simulink library "Pipe_BiFlow"  (R2018b)
settings: Solver=ode45  StartTime=0.0  StopTime=10.0  RelTol=1e-3  EnableMultiTasking=on
undefined symbols (not defined in the file): path_carnot
libraries: carnot x5
settings Model: Creator=drhf  LastModifiedBy=P41573
settings DataIOCC: LimitDataPoints=on  SaveFormat=Array  SignalLoggingSaveFormat=ModelDataLogs
settings OptimizationCC: ExpressionDepthLimit=2147483647  LifeSpan=inf
settings DebuggingCC: UnderspecifiedInitializationDetection=Classic  MergeDetectMultiDrivingBlocksExec=none  SolverPrmCheckMsg=warning  FcnCallInpInsideContextMsg=warning  StateNameClashWarn=warning  SFUnexpectedBacktrackingDiag=warning  SFNoUnconditionalDefaultTransitionDiag=warning  SFExecutionAtInitializationDiag=none
settings HardwareCC: ProdBitPerPointer=32  ProdBitPerSizeT=32  ProdBitPerPtrDiffT=32  ProdLargestAtomicFloat=None  ProdIntDivRoundTo=Undefined  ProdEndianess=Unspecified  ProdWordSize=32  ProdHWDeviceType=32-bit Generic
settings ModelReferenceCC: PropagateSignalLabelsOutOfModel=off
settings SFSimCC: SimUseLocalCustomCode=off
settings RTWCC: RTWUseLocalCustomCode=off
settings CodeAppCC: StateflowObjectComments=on
settings GRTTargetCC: TargetLangStandard=C89/C90 (ANSI)  GeneratePreprocessorConditionals=Disable all  CombineOutputUpdateFcns=off  GRTInterface=on
settings ConfigComp: CovMetricSettings=dw  CovHtmlReporting=on  CovSaveCumulativeToWorkspaceVar=on  CovSaveSingleToWorkspaceVar=on  CovExternalEMLEnable=off

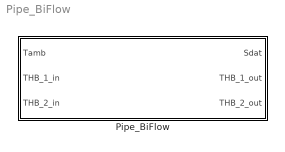
== system Pipe_BiFlow ==
  Pipe_BiFlow : Subsystem  mask(Pipe Biflow){t0=20, hgt=1273.2395, stgtype=1, tini=[20 20 20 20 20 20 20 20 20 20], mpts=[1 2 3 4 5 6 7 8 9 10], PathName=fullfile(path_carnot('libsl'),'Hydraulics','Pipe_BiFlow','parameter_set'), FileName='PipeBF_set1.mat', userPath=off, userParam=off, uwall=1, ubot=0, utop=0, axcond=1, volume=10, dia=0.1, standing=standing cylinder, nodes=10, mpoints=10, pipe1inlet=1, pipe1outlet=0, pipe1dia=0.1, pipe2inlet=0, pipe2outlet=1, pipe2dia=0.1}
      mask prompts: t0 "Initial temperature (vector or scalar) in °C"; hgt "Length of pipe in m"; stgtype "Storage Type (0..5)"; tini "Start temperatures of nodes in °C"; mpts "Index to measured nodes"; PathName "Path"; FileName "Parameter set"; userPath "Edit path and name of parameter set"; userParam "User defined parameters"; uwall "Heat transfer coefficient to ambient [W/m²K]"; ubot "Heat transfer coefficient to ambient bottom [W/m²K]"; utop "Heat transfer coefficient to ambient top [W/m²K]"; axcond "Effective thermal conductivity [W/m/K]"; volume "Volume [m³]"; dia "Diameter [m]"; standing "Position"; nodes "Number of nodes"; mpoints "Number of node temperatures (for display)"; pipe1inlet "relative height of inlet, range from 0 (= bottom) to 1 (= top)"; pipe1outlet "relative height of outlet, range from 0 (= bottom) to 1 (= top)"; pipe1dia "Diameter of connection in m"; pipe2inlet "relative height of inlet, range from 0 (= bottom) to 1 (= top)"; pipe2outlet "relative height of outlet, range from 0 (= bottom) to 1 (= top)"; pipe2dia "Diameter of connection in m"
      mask help: Pipe model for flow in both directions. The model is based on a buffer storage tank but has no calculation for inversed thermocline.
      mask init:
      | [ok, param] = CarnotCallbacks_PipeBiflow('SetParam',1,gcbh,PathName,FileName);
      mask Help: web(fullfile(path_carnot('help'),'PipeBilfow.html'),'-helpbrowser')
      mask TypeOptions hgt: Pipe_Connection_1/hgt | Pipe_Connection_2/hgt
      mask TypeOptions stgtype: CreateSdat/stgtype
      mask TypeOptions tini: sfun_storageTnodes/tini
      mask TypeOptions mpts: select_T/Indices
      mask Callback userPath: [ok, param] = CarnotCallbacks_StorageConf('UserEdit',1,gcbh);
      mask Callback userParam: [ok, param] = CarnotCallbacks_StorageConf('UserEdit',1,gcbh);
      mask TypeOptions uwall: sfun_storageTnodes/uloss
      mask TypeOptions ubot: sfun_storageTnodes/ubot
      mask TypeOptions utop: sfun_storageTnodes/utop
      mask TypeOptions axcond: sfun_storageTnodes/cond
      mask TypeOptions volume: sfun_storageTnodes/volume | CreateSdat/volume
      mask TypeOptions dia: sfun_storageTnodes/dia | Pipe_Connection_1/dstg | Pipe_Connection_2/dstg
      mask TypeOptions standing: sfun_storageTnodes/standing
      mask TypeOptions nodes: sfun_storageTnodes/nodes | select_T/InputPortWidth | HX_EN12977_1/nodes | HX_EN12977_2/nodes | HX_EN12977_3/nodes | Pipe_Connection_1/nodes | Pipe_Connection_2/nodes | Pipe_Connection_3/nodes
      mask TypeOptions pipe1inlet: Pipe_Connection_1/h_in
      mask TypeOptions pipe1outlet: Pipe_Connection_1/h_out
      mask TypeOptions pipe1dia: Pipe_Connection_1/dpipe
      mask TypeOptions pipe2inlet: Pipe_Connection_2/h_in
      mask TypeOptions pipe2outlet: Pipe_Connection_2/h_out
      mask TypeOptions pipe2dia: Pipe_Connection_2/dpipe
      mask DialogControl Container14 Prompt: Infos
      mask DialogControl ParameterGroupVar Prompt: Picking a parameter set
      mask DialogControl Control3 Prompt: Carnot public data
      mask DialogControl Control3 Callback: [ok, file] = CarnotCallbacks_PipeBiflow('GetFilename',1,gcbh,'public');
      mask DialogControl Control4 Prompt: Carnot internal data
      mask DialogControl Control4 Callback: [ok, file] = CarnotCallbacks_PipeBiflow('GetFilename',1,gcbh,'internal');
      mask DialogControl Control2 Prompt: Selected path
      mask DialogControl Control2 Callback: [ok, file] = CarnotCallbacks_PipeBiflow('GetFilename',1,gcbh,'selected');
      mask DialogControl Container4 Prompt: Parameter values
      mask DialogControl Container6 Prompt: Pipe
      mask DialogControl Container8 Prompt: Connections
      mask DialogControl Container9 Prompt: Inlet 1
      mask DialogControl Container12 Prompt: Inlet 2
      mask DialogControl Control6 Prompt: Save in Carnot internal data
      mask DialogControl Control6 Callback: [ok, param] = CarnotCallbacks_PipeBiflow('SaveFilename',1,gcbh,'internal','PipeBF');
      mask DialogControl Control5 Prompt: Save in selected path
      mask DialogControl Control5 Callback: [ok, param] = CarnotCallbacks_PipeBiflow('SaveFilename',1,gcbh,'selected','PipeBF');
      mask Display:
      | % user defined picture file
      | picfile = fullfile(path_carnot('intlibsl'), 'Hydraulics','Pipe_Biflow', ...
      |     'parameter_set', 'Pipe_Biflow.jpg');
      | 
      | % show internal picture if defined
      | pic = false;
      | if  ~BlockIsInCarnotLibrary       % if not located in library
      |     if exist(picfile, 'file')
      |         image(imread(picfile), [0.25, 0, 0.45, 1])
      |         set_param(gcb, 'BackgroundColor', 'White')
      |         pic = true;
      |     end
      | end
      | 
      | % show public picture
      | if ~pic
      |     set_param(gcb, 'BackgroundColor', 'Red')
      |     plot(0,0,1,1,[24,27,27,24,75,80,80,75,24,20,20,24]/100,[60,53,46,40,40,46,55,60,60,53,46,40]/100)
      | end

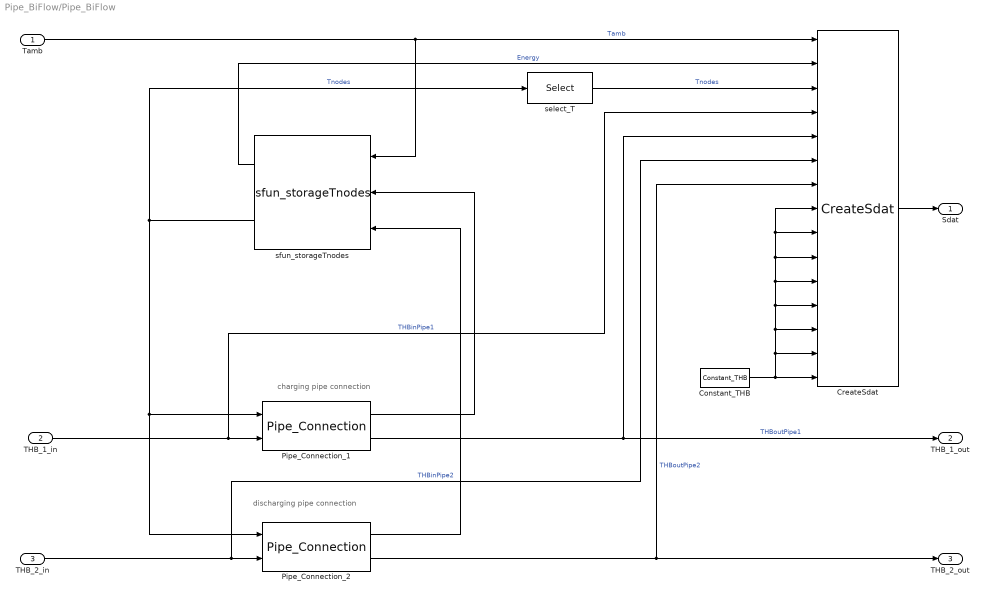
== system Pipe_BiFlow/Pipe_BiFlow ==
  note: charging pipe connection
  note: discharging pipe connection
  Tamb : Inport
  THB_1_in : Inport  Port=2
  THB_2_in : Inport  Port=3
  Constant_THB : carnot/Source/Simple/Constant_THB  t=20  mdot=0  p=1e5  mID=No Pressure Drop  fluid=Water  mix=0  mix2=0  mix3=0  dia=0.02  hgt=0
      settings: SourceProductName=Carnot
  CreateSdat : carnot/Basic/Thermal_Models/CreateSdat  volume=volume  stgtype=stgtype
      settings: SourceProductName=Carnot
  Pipe_Connection_1 : carnot/Storage/Thermal/Storage_Ports/Pipe_Connection  h_in=pipe1inlet  h_out=pipe1outlet  hgt=hgt  dpipe=pipe1dia  dstg=dia  height=-1273.2395  nodes=nodes
      settings: SourceProductName=Carnot
  Pipe_Connection_2 : carnot/Storage/Thermal/Storage_Ports/Pipe_Connection  h_in=pipe2inlet  h_out=pipe2outlet  hgt=hgt  dpipe=pipe2dia  dstg=dia  height=1273.2395  nodes=nodes
      settings: SourceProductName=Carnot
  select_T : Selector  InputPortWidth=nodes  IndexOptions=Index vector (dialog)  Indices=[1 2 3 4 5 6 7 8 9 10]  OutputSizes=1
  sfun_storageTnodes : carnot/Basic/Thermal_Models/sfun_storageTnodes  uloss=uwall  ubot=ubot  utop=utop  cond=axcond  volume=volume  dia=dia  standing=standing cylinder  tini=tini  nodes=nodes  nconnect=2  elimthermocline=0  condinvtc=0
      settings: SourceProductName=Carnot
  Sdat : Outport
  THB_1_out : Outport  Port=2
  THB_2_out : Outport  Port=3
  wires:
  sfun_storageTnodes/1 -> CreateSdat/2  "Energy"
  Pipe_Connection_2/2 -> CreateSdat/7, THB_2_out/1  "THBoutPipe2"
  Pipe_Connection_2/1 -> sfun_storageTnodes/3
  THB_2_in/1 -> Pipe_Connection_2/2, CreateSdat/6  "THBinPipe2"
  Tamb/1 -> sfun_storageTnodes/1, CreateSdat/1  "Tamb"
  select_T/1 -> CreateSdat/3  "Tnodes"
  sfun_storageTnodes/2 -> Pipe_Connection_2/1, Pipe_Connection_1/1, select_T/1  "Tnodes"
  CreateSdat/1 -> Sdat/1
  THB_1_in/1 -> CreateSdat/4, Pipe_Connection_1/2  "THBinPipe1"
  Pipe_Connection_1/2 -> CreateSdat/5, THB_1_out/1  "THBoutPipe1"
  Pipe_Connection_1/1 -> sfun_storageTnodes/2
  Constant_THB/1 -> CreateSdat/14, CreateSdat/13, CreateSdat/12, CreateSdat/11, CreateSdat/10, CreateSdat/9, CreateSdat/8, CreateSdat/15
